simulink subsystem "Attitude_controller"  (R2020a)
settings: Solver=VariableStepAuto  StartTime=0.0  StopTime=10.0  RelTol=1e-3
settings Model: Creator=decla  LastModifiedBy=decla

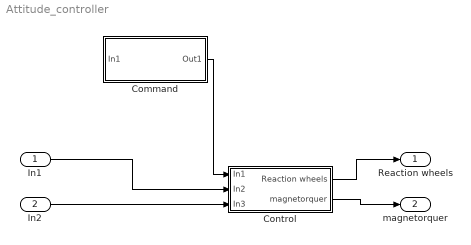
== system Attitude_controller ==
  In1 : Inport
  In2 : Inport  Port=2
  Command : Subsystem
  Control : Subsystem
  Reaction wheels : Outport
  magnetorquer : Outport  Port=2
  wires:
  Command/1(Out1) -> Control/1(In1)
  Control/1(Reaction wheels) -> Reaction wheels/1
  Control/2(magnetorquer) -> magnetorquer/1
  In1/1 -> Control/2(In2)
  In2/1 -> Control/3(In3)

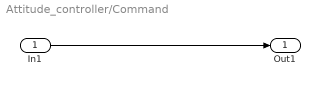
== system Attitude_controller/Command ==
  In1 : Inport
  Out1 : Outport
  wires:
  In1/1 -> Out1/1

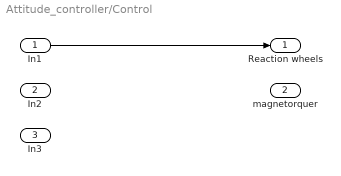
== system Attitude_controller/Control ==
  In1 : Inport
  In2 : Inport  Port=2
  In3 : Inport  Port=3
  Reaction wheels : Outport
  magnetorquer : Outport  Port=2
  wires:
  In1/1 -> Reaction wheels/1
